simulink model "IV_actividad2"  (Simulink 7.9)
settings: Solver=ode45  StartTime=0.0  StopTime=2500.0  RelTol=1e-3
undefined symbols (not defined in the file or in its folder): ctrl, Kd, Ki, Kp, lambda
libraries: nintblocks x2
settings Model: Creator=root  LastModifiedBy=root
settings DebuggingCC: MaxConsecutiveZCsMsg=warning

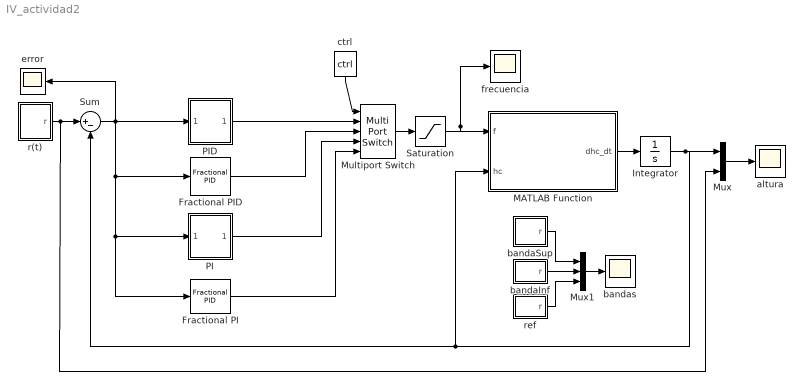
== system IV_actividad2 ==
  Fractional PI : nintblocks/Fractional PID  kp=Kp  kd=Kd  vd=mu  ki=Ki  vi=-lambda  bandwidth=[0.01 100]  n=100  form1=crone  exp1=mcltime  decomp1=frac
  Fractional PID : nintblocks/Fractional PID  kp=Kp  kd=Kd  vd=mu  ki=Ki  vi=-lambda  bandwidth=[0.01 100]  n=100  form1=crone  exp1=mcltime  decomp1=frac
  Integrator : Integrator  InitialCondition=10  UpperSaturationLimit=70  LowerSaturationLimit=0
  MATLAB Function : MATLAB Function  TreatAsAtomicUnit=on
  Multiport Switch : MultiPortSwitch  Inputs=4  zeroidx=off
  Mux : Mux  Inputs=2
  Mux1 : Mux  Inputs=3
  PI : Subsystem
  PID : Subsystem
  Saturation : Saturate  UpperLimit=100  LowerLimit=0
  Sum : Sum  Inputs=|+-
  altura : Scope
      settings: TimeRange=971.6614906832298  YMin=13  YMax=22.5  SaveName=hc
  bandaInf : Subsystem
  bandaSup : Subsystem
  bandas : Scope
      settings: TimeRange=971.6614906832298  YMin=14.5  YMax=22.5  SaveName=bandas
  ctrl : Constant  Value=ctrl
  error : Scope
      settings: SaveName=error
  frecuencia : Scope
      settings: SaveName=salidaControlador
  r(t) : Subsystem
  ref : Subsystem
  wires:
  Integrator/1 -> MATLAB Function/2(hc), Sum/2, Mux/1
  Sum/1 -> error/1, PID/1(In1), Fractional PID/1, Fractional PI/1, PI/1(In1)
  r(t)/1(r) -> Sum/1, Mux/2
  Saturation/1 -> frecuencia/1, MATLAB Function/1(f)
  MATLAB Function/1(dhc_dt) -> Integrator/1
  Mux/1 -> altura/1
  Multiport Switch/1 -> Saturation/1
  PID/1(Out1) -> Multiport Switch/2
  Fractional PID/1 -> Multiport Switch/3
  PI/1(Out1) -> Multiport Switch/4
  Fractional PI/1 -> Multiport Switch/5
  ctrl/1 -> Multiport Switch/1
  Mux1/1 -> bandas/1
  bandaSup/1(r) -> Mux1/1
  bandaInf/1(r) -> Mux1/2
  ref/1(r) -> Mux1/3

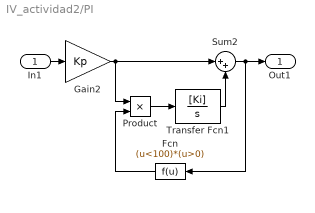
== system IV_actividad2/PI ==
  In1 : Inport
  Fcn : Fcn  Expr=(u<100)*(u>0)
  Gain2 : Gain  Gain=Kp
  Product : Product  RndMeth=Zero
  Sum2 : Sum  Inputs=|++
  Transfer Fcn1 : TransferFcn  Numerator=[Ki]  Denominator=[1 0]
  Out1 : Outport
  wires:
  Gain2/1 -> Sum2/1, Product/1
  Sum2/1 -> Fcn/1, Out1/1
  Transfer Fcn1/1 -> Sum2/2
  Product/1 -> Transfer Fcn1/1
  Fcn/1 -> Product/2
  In1/1 -> Gain2/1

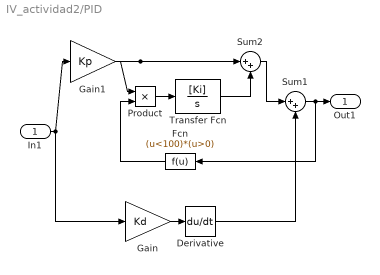
== system IV_actividad2/PID ==
  In1 : Inport
  Derivative : Derivative
  Fcn : Fcn  Expr=(u<100)*(u>0)
  Gain : Gain  Gain=Kd
  Gain1 : Gain  Gain=Kp
  Product : Product  RndMeth=Zero
  Sum1 : Sum  Inputs=|++
  Sum2 : Sum  Inputs=|++
  Transfer Fcn : TransferFcn  Numerator=[Ki]  Denominator=[1 0]
  Out1 : Outport
  wires:
  Gain/1 -> Derivative/1
  Gain1/1 -> Sum2/1, Product/1
  Sum2/1 -> Sum1/1
  Transfer Fcn/1 -> Sum2/2
  Product/1 -> Transfer Fcn/1
  Fcn/1 -> Product/2
  In1/1 -> Gain/1, Gain1/1
  Sum1/1 -> Out1/1, Fcn/1
  Derivative/1 -> Sum1/2

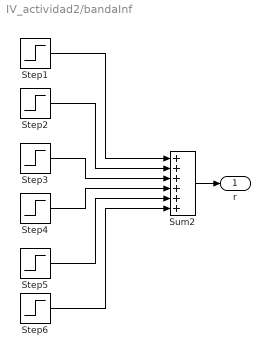
== system IV_actividad2/bandaInf ==
  Step1 : Step  Time=400  Before=22.5*0.98  After=22.5*0.98  SampleTime=0
  Step2 : Step  Time=401  After=15*0.98
  Step3 : Step  Time=801  After=15*0.98
  Step4 : Step  Time=1201  After=-15*0.98
  Step5 : Step  Time=1601  After=-15*0.98
  Step6 : Step  Time=2001  After=-7.5*0.98
  Sum2 : Sum  Inputs=++++++
  r : Outport
  wires:
  Sum2/1 -> r/1
  Step1/1 -> Sum2/1
  Step2/1 -> Sum2/2
  Step5/1 -> Sum2/5
  Step6/1 -> Sum2/6
  Step3/1 -> Sum2/3
  Step4/1 -> Sum2/4

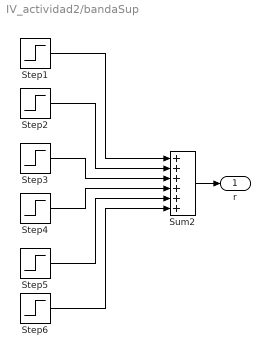
== system IV_actividad2/bandaSup ==
  Step1 : Step  Time=400  Before=22.5*(1.02)  After=22.5*(1.02)  SampleTime=0
  Step2 : Step  Time=401  After=15*(1.02)
  Step3 : Step  Time=801  After=15*(1.02)
  Step4 : Step  Time=1201  After=-15*(1.02)
  Step5 : Step  Time=1601  After=-15*(1.02)
  Step6 : Step  Time=2001  After=-7.5*(1.02)
  Sum2 : Sum  Inputs=++++++
  r : Outport
  wires:
  Sum2/1 -> r/1
  Step1/1 -> Sum2/1
  Step2/1 -> Sum2/2
  Step5/1 -> Sum2/5
  Step6/1 -> Sum2/6
  Step3/1 -> Sum2/3
  Step4/1 -> Sum2/4

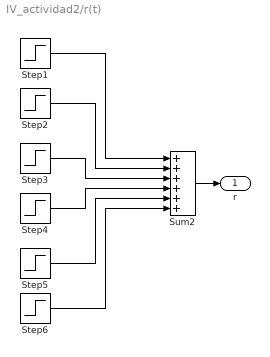
== system IV_actividad2/r(t) ==
  Step1 : Step  Time=400  Before=22.5  After=22.5  SampleTime=0
  Step2 : Step  Time=401  After=15
  Step3 : Step  Time=801  After=15
  Step4 : Step  Time=1201  After=-15
  Step5 : Step  Time=1601  After=-15
  Step6 : Step  Time=2001  After=-7.5
  Sum2 : Sum  Inputs=++++++
  r : Outport
  wires:
  Sum2/1 -> r/1
  Step1/1 -> Sum2/1
  Step2/1 -> Sum2/2
  Step5/1 -> Sum2/5
  Step6/1 -> Sum2/6
  Step3/1 -> Sum2/3
  Step4/1 -> Sum2/4

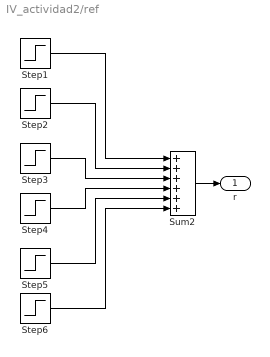
== system IV_actividad2/ref ==
  Step1 : Step  Time=400  Before=22.5  After=22.5  SampleTime=0
  Step2 : Step  Time=401  After=15
  Step3 : Step  Time=801  After=15
  Step4 : Step  Time=1201  After=-15
  Step5 : Step  Time=1601  After=-15
  Step6 : Step  Time=2001  After=-7.5
  Sum2 : Sum  Inputs=++++++
  r : Outport
  wires:
  Sum2/1 -> r/1
  Step1/1 -> Sum2/1
  Step2/1 -> Sum2/2
  Step5/1 -> Sum2/5
  Step6/1 -> Sum2/6
  Step3/1 -> Sum2/3
  Step4/1 -> Sum2/4

== matlab function MATLAB Function ==
  data: f input double; dhc_dt output double; hc input double
function dhc_dt = ModeloNoLineal(f, hc)
%#codegen

    dhc_dt = (5.43*f-78.43-20.21*sqrt(abs(hc)))/(0.63*(hc.^2)+11.4*hc+17.1);
end
